simulink model "ASR_3rd4thSaturation_10_Disturb"  (R2020a)
settings: Solver=ode45  StartTime=0.0  StopTime=50.0  MaxStep=1e-5  RelTol=1e-3
settings Model: Creator=78253  LastModifiedBy=78253

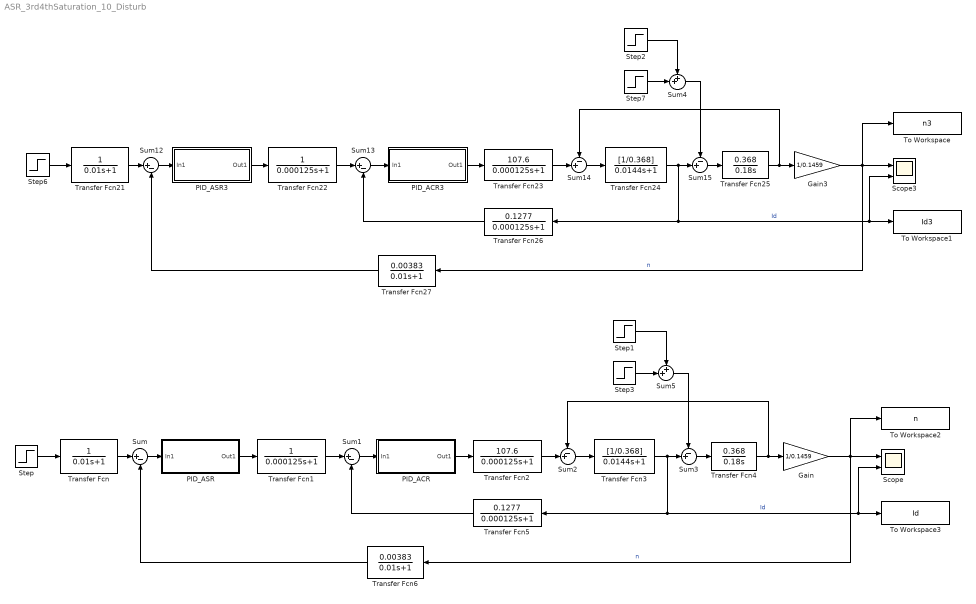
== system ASR_3rd4thSaturation_10_Disturb ==
  Gain : Gain  Gain=1/0.1459
  Gain3 : Gain  Gain=1/0.1459
  PID_ACR : Subsystem
  PID_ACR3 : Subsystem
  PID_ASR : Subsystem
  PID_ASR3 : Subsystem
  Scope : Scope  NumInputPorts=2
  Scope3 : Scope  NumInputPorts=2
  Step : Step  Time=0  After=10  SampleTime=0
  Step1 : Step  Time=20  After=20  SampleTime=0
  Step2 : Step  Time=20  After=20  SampleTime=0
  Step3 : Step  Time=0  After=52.2  SampleTime=0
  Step6 : Step  Time=0  After=10  SampleTime=0
  Step7 : Step  Time=0  After=52.2  SampleTime=0
  Sum{,1,12..13} (4 alike) : Sum  Inputs=|+-
  Sum{2..3,14..15} (4 alike) : Sum  Inputs=-+|
  Sum4 : Sum  Inputs=++|
  Sum5 : Sum  Inputs=++|
  To Workspace : ToWorkspace  VariableName=n3  SaveFormat=Timeseries  SampleTime=-1
  To Workspace1 : ToWorkspace  VariableName=Id3  SaveFormat=Timeseries  SampleTime=-1
  To Workspace2 : ToWorkspace  VariableName=n  SaveFormat=Timeseries  SampleTime=-1
  To Workspace3 : ToWorkspace  VariableName=Id  SaveFormat=Timeseries  SampleTime=-1
  Transfer Fcn : TransferFcn  Denominator=[0.01 1]
  Transfer Fcn1 : TransferFcn  Denominator=[0.000125 1]
  Transfer Fcn2 : TransferFcn  Numerator=[107.6]  Denominator=[0.000125 1]
  Transfer Fcn21 : TransferFcn  Denominator=[0.01 1]
  Transfer Fcn22 : TransferFcn  Denominator=[0.000125 1]
  Transfer Fcn23 : TransferFcn  Numerator=[107.6]  Denominator=[0.000125 1]
  Transfer Fcn24 : TransferFcn  Numerator=[1/0.368]  Denominator=[0.0144 1]
  Transfer Fcn25 : TransferFcn  Numerator=[0.368]  Denominator=[0.18 0]
  Transfer Fcn26 : TransferFcn  Numerator=[0.1277]  Denominator=[0.000125 1]
  Transfer Fcn27 : TransferFcn  Numerator=[0.00383]  Denominator=[0.01 1]
  Transfer Fcn3 : TransferFcn  Numerator=[1/0.368]  Denominator=[0.0144 1]
  Transfer Fcn4 : TransferFcn  Numerator=[0.368]  Denominator=[0.18 0]
  Transfer Fcn5 : TransferFcn  Numerator=[0.1277]  Denominator=[0.000125 1]
  Transfer Fcn6 : TransferFcn  Numerator=[0.00383]  Denominator=[0.01 1]
  wires:
  Transfer Fcn21/1 -> Sum12/1
  PID_ACR3/1(Out1) -> Transfer Fcn23/1
  Transfer Fcn23/1 -> Sum14/2
  Sum13/1 -> PID_ACR3/1(In1)
  Step6/1 -> Transfer Fcn21/1
  Transfer Fcn22/1 -> Sum13/1
  PID_ASR/1(Out1) -> Transfer Fcn1/1
  Transfer Fcn27/1 -> Sum12/2
  Sum1/1 -> PID_ACR/1(In1)
  Transfer Fcn26/1 -> Sum13/2
  Transfer Fcn25/1 -> Sum14/1, Gain3/1
  Sum2/1 -> Transfer Fcn3/1
  Sum14/1 -> Transfer Fcn24/1
  Transfer Fcn24/1 -> Transfer Fcn26/1, To Workspace1/1, Scope3/2, Sum15/2  "Id"
  Sum12/1 -> PID_ASR3/1(In1)
  Transfer Fcn6/1 -> Sum/2
  Gain/1 -> To Workspace2/1, Transfer Fcn6/1, Scope/1  "n"
  Transfer Fcn3/1 -> Transfer Fcn5/1, To Workspace3/1, Scope/2, Sum3/2  "Id"
  Sum15/1 -> Transfer Fcn25/1
  Sum/1 -> PID_ASR/1(In1)
  Transfer Fcn5/1 -> Sum1/2
  PID_ASR3/1(Out1) -> Transfer Fcn22/1
  Transfer Fcn2/1 -> Sum2/2
  Step/1 -> Transfer Fcn/1
  Transfer Fcn4/1 -> Sum2/1, Gain/1
  PID_ACR/1(Out1) -> Transfer Fcn2/1
  Gain3/1 -> To Workspace/1, Transfer Fcn27/1, Scope3/1  "n"
  Transfer Fcn/1 -> Sum/1
  Sum3/1 -> Transfer Fcn4/1
  Transfer Fcn1/1 -> Sum1/1
  Step7/1 -> Sum4/2
  Sum4/1 -> Sum15/1
  Step2/1 -> Sum4/1
  Sum5/1 -> Sum3/1
  Step3/1 -> Sum5/2
  Step1/1 -> Sum5/1

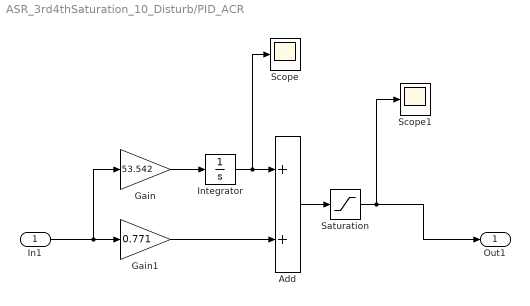
== system ASR_3rd4thSaturation_10_Disturb/PID_ACR ==
  In1 : Inport
  Add : Sum
  Gain : Gain  Gain=53.542
  Gain1 : Gain  Gain=0.771
  Integrator : Integrator  LimitOutput=on  UpperSaturationLimit=5  LowerSaturationLimit=-5
  Saturation : Saturate  UpperLimit=5  LowerLimit=-5
  Scope : Scope
  Scope1 : Scope
  Out1 : Outport
  wires:
  In1/1 -> Gain/1, Gain1/1
  Gain1/1 -> Add/2
  Add/1 -> Saturation/1
  Gain/1 -> Integrator/1
  Saturation/1 -> Out1/1, Scope1/1
  Integrator/1 -> Scope/1, Add/1

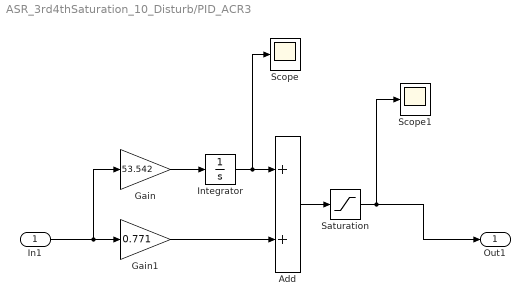
== system ASR_3rd4thSaturation_10_Disturb/PID_ACR3 ==
  In1 : Inport
  Add : Sum
  Gain : Gain  Gain=53.542
  Gain1 : Gain  Gain=0.771
  Integrator : Integrator  LimitOutput=on  UpperSaturationLimit=5  LowerSaturationLimit=-5
  Saturation : Saturate  UpperLimit=5  LowerLimit=-5
  Scope : Scope
  Scope1 : Scope
  Out1 : Outport
  wires:
  In1/1 -> Gain/1, Gain1/1
  Gain1/1 -> Add/2
  Add/1 -> Saturation/1
  Gain/1 -> Integrator/1
  Saturation/1 -> Out1/1, Scope1/1
  Integrator/1 -> Scope/1, Add/1

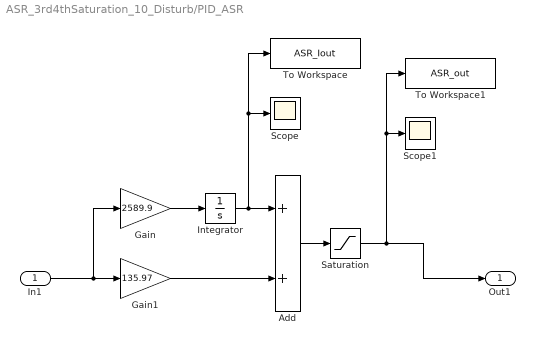
== system ASR_3rd4thSaturation_10_Disturb/PID_ASR ==
  In1 : Inport
  Add : Sum
  Gain : Gain  Gain=2589.9
  Gain1 : Gain  Gain=135.97
  Integrator : Integrator  LimitOutput=on  UpperSaturationLimit=10  LowerSaturationLimit=-10
  Saturation : Saturate  UpperLimit=10  LowerLimit=-10
  Scope : Scope
  Scope1 : Scope
  To Workspace : ToWorkspace  VariableName=ASR_Iout  SaveFormat=Timeseries  SampleTime=-1
  To Workspace1 : ToWorkspace  VariableName=ASR_out  SaveFormat=Timeseries  SampleTime=-1
  Out1 : Outport
  wires:
  In1/1 -> Gain/1, Gain1/1
  Gain/1 -> Integrator/1
  Gain1/1 -> Add/2
  Integrator/1 -> To Workspace/1, Scope/1, Add/1
  Add/1 -> Saturation/1
  Saturation/1 -> To Workspace1/1, Scope1/1, Out1/1

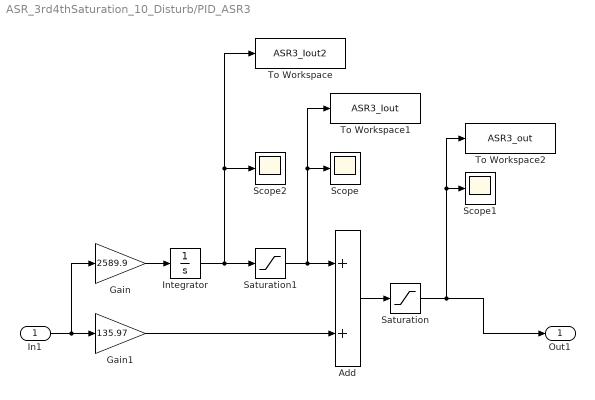
== system ASR_3rd4thSaturation_10_Disturb/PID_ASR3 ==
  In1 : Inport
  Add : Sum
  Gain : Gain  Gain=2589.9
  Gain1 : Gain  Gain=135.97
  Integrator : Integrator  UpperSaturationLimit=10  LowerSaturationLimit=-10
  Saturation : Saturate  UpperLimit=10  LowerLimit=-10
  Saturation1 : Saturate  UpperLimit=10  LowerLimit=-10
  Scope : Scope
  Scope1 : Scope
  Scope2 : Scope
  To Workspace : ToWorkspace  VariableName=ASR3_Iout2  SaveFormat=Timeseries  SampleTime=-1
  To Workspace1 : ToWorkspace  VariableName=ASR3_Iout  SaveFormat=Timeseries  SampleTime=-1
  To Workspace2 : ToWorkspace  VariableName=ASR3_out  SaveFormat=Timeseries  SampleTime=-1
  Out1 : Outport
  wires:
  In1/1 -> Gain1/1, Gain/1
  Gain1/1 -> Add/2
  Add/1 -> Saturation/1
  Saturation/1 -> Scope1/1, To Workspace2/1, Out1/1
  Gain/1 -> Integrator/1
  Saturation1/1 -> Scope/1, To Workspace1/1, Add/1
  Integrator/1 -> Saturation1/1, To Workspace/1, Scope2/1
